simulink library "vhit_control_library"  (R2023a)
settings: Solver=VariableStepAuto  StartTime=0.0  StopTime=10.0  RelTol=1e-3
undefined symbols (not defined in the file): bit, cstElctSpdMaxVal, cstSlowTaskSampTime, parDirCurrMaxVal, parElctSpdMaxVal, parFluxObsFiltCoef, parQdrtCurrMaxVal, parRefSpdFallSlewRate, parRefSpdRisSlewRate, PolePairNum
libraries: lib_conversion x90, lib_square_root x11, lib_dynamic_saturator x9, lib_resettable_unit_delay x2, lib_fault_definiteness x1, lib_angle_mapper x1, lib_cart_to_polar_coor_transformer x1, lib_clarke_transform x1, lib_configurable_parameter x1, lib_current_control_decoupling x1, lib_derating_reference_speed_limiter x1, lib_discrete_time_integrator x1
(part 1 of 3)
settings Model: Creator=CAV2OFO  LastModifiedBy=xiaoqiang.yuan
settings SolverCC: AlgebraicLoopSolver=TrustRegion
settings OptimizationCC: ReuseModelBlockBuffer=off
settings DebuggingCC: UnconnectedInputMsg=warning  UnconnectedOutputMsg=warning  UnconnectedLineMsg=warning
settings ModelReferenceCC: EnableRefExpFcnMdlSchedulingChecks=on
settings RTWCC: DLArmComputeVersion=19.05

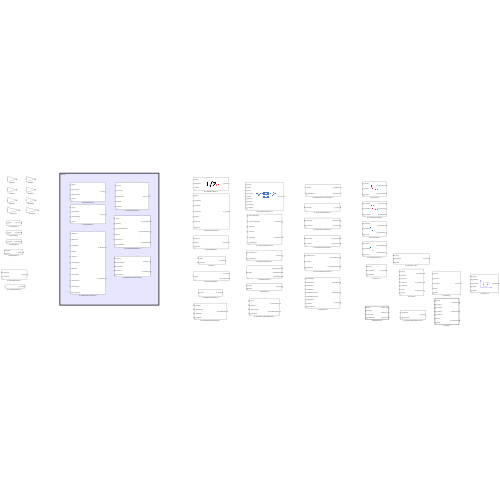
[thumbnail: Simulink's stored preview of the top-level diagram]
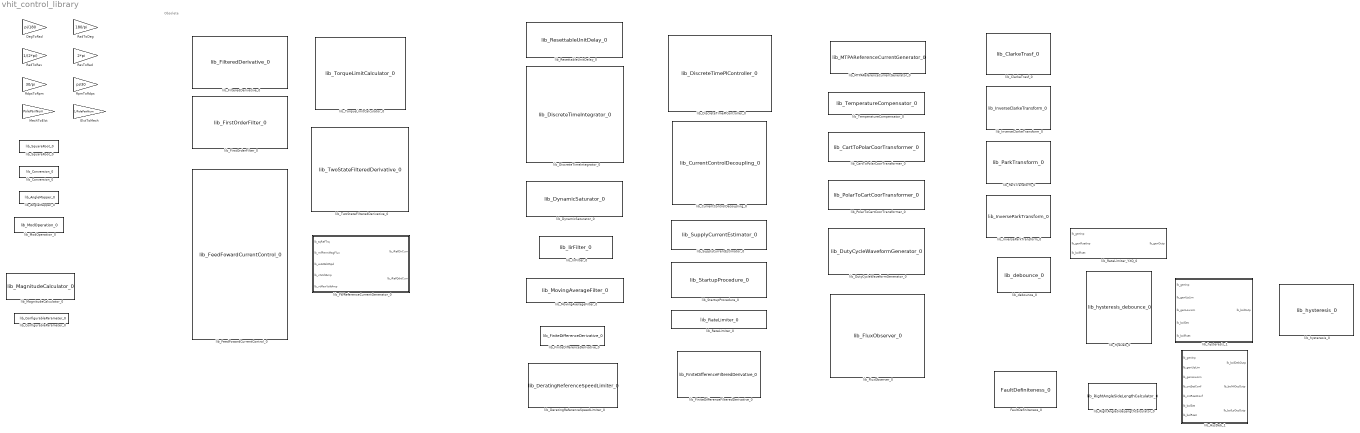
== system vhit_control_library ==
  note: Obsolete
  DegToRad : Gain  Gain=pi/180
  ElctToMech : Gain  Gain=1/PolePairNum
  FaultDefiniteness_0 : lib_fault_definiteness/FaultDefiniteness_0  lb_FaltWaitRecvCnt=0
      link override Constant0: Value=lb_FailWaitRecvCnt
  MechToElct : Gain  Gain=PolePairNum
  RadToDeg : Gain  Gain=180/pi
  RadToRev : Gain  Gain=1/(2*pi)
  RdpsToRpm : Gain  Gain=30/pi
  RevToRad : Gain  Gain=2*pi
  RpmToRdps : Gain  Gain=pi/30
  lib_AngleMapper_0 : lib_angle_mapper/lib_AngleMapper_0  lb_parSlctMappMode=[0,4pi] to [0,2pi]  lb_parOutpDataType=Inherit: Inherit via back propagation
  lib_CartToPolarCoorTransformer_0 : lib_cart_to_polar_coor_transformer/lib_CartToPolarCoorTransformer_0  lb_parAsinLktSize=4095  lb_parAmpLktSize=512  lb_parOutpAmpDataType=fixdt(0,16,2^-10,0)
  lib_ClarkeTrasf_0 : lib_clarke_transform/lib_ClarkeTrasf_0  VariantControl=ClarkTransf_MIL_flo  lb_parAccmDataType=fixdt(1,16,2^-6,0)  lb_parUnBalcSys=off
  lib_ConfigurableParameter_0 : lib_configurable_parameter/lib_ConfigurableParameter_0  lb_parCnfgPar=1  lb_parDataType=Inherit: Inherit from 'Constant value'  lb_parUpLim=2  lb_parLowLim=0
  lib_Conversion_0 : lib_conversion/lib_Conversion_0  lb_parDataType=Inherit: Inherit via back propagation  lb_parOutpMaxVal=[]  lb_parOutpMinVal=[]  lb_parSatFlag=off
  lib_CurrentControlDecoupling_0 : lib_current_control_decoupling/lib_CurrentControlDecoupling_0  lb_parDirIndc=0  lb_parQdrtIndc=0  lb_parMaxPhsIndc=0.001  lb_parMaxElctSpd=4096  lb_parMaxPhsCurr=100  lb_parMaxPermMagFlux=0.01  lb_parMaxCtrlPhsVolt=40  lb_parOutpPekPhy=64  lb_parOutpDataType=fixdt(1,16,2^0,0)
  lib_DeratingReferenceSpeedLimiter_0 : lib_derating_reference_speed_limiter/lib_DeratingReferenceSpeedLimiter_0  lb_parSampTime=parSlowTaskSampTime_u16d6b0  lb_parMaxSampTime=0.01  lb_parMaxIntgGain=parRefSpdLimIntgGainMaxVal  lb_parMaxCurrMarg=100  lb_parMinCurrMarg=-1  lb_parMaxElctRefSpd=2600  lb_parIntgScopMode=Integral control  lb_parSatFlag=on  lb_parAccmDataTypeMode=16-bit  lb_parDtiAccmDataTypeMode=Same of output  lb_parRefSpdDataType=fixdt(1,16,2^-3,0)
  lib_DiscreteTimeIntegrator_0 : lib_discrete_time_integrator/lib_DiscreteTimeIntegrator_0  lb_parMaxInpVal=1  lb_parMinInpVal=-1  lb_parMaxSampTime=0.01  lb_parMaxIntgGain=0  lb_parAccmDataTypeMode=Same of output  lb_parOutpDataType=fixdt(1,16,2^-3,0)  lb_parIntgScopMode=Generic signal  lb_parSatFlag=off
  lib_DiscreteTimePIController_0 : lib_discrete_time_PI_controller/lib_DiscreteTimePIController_0  lb_parSampTime=0.01  lb_parMaxSampTime=1  lb_parMaxPropGain=1  lb_parMaxIntgGain=1  lb_parRefInpMaxVal=4096  lb_parRefInpMinVal=-4096  lb_parMaxErrVal=4096*2  lb_parMinErrVal=-4096*2  lb_parMaxOutpVal=20  lb_parMinOutpVal=-20  lb_parAccmDataTypeMode=32-bit  lb_parOutpDataType=fixdt(1,16,2^-14,0)  lb_parSatMode=anti-windup with back-calculation
  lib_DutyCycleWaveformGenerator_0 : lib_duty_cycle_waveform_generator/lib_DutyCycleWaveformGenerator_0  lb_parLktSize=1024  lb_parOmodFact=1  lb_parPWMMode=Sinusoidal plus third harmonics modulation
  lib_DynamicSaturator_0 : lib_dynamic_saturator/lib_DynamicSaturator_0
  lib_FWReferenceCurrentGenerator_0 : Subsystem  mask{lb_parPolePairNum=5, lb_parPermMagFlux=2e-3, lb_parMagTempCoef=-1e-3, lb_parDirIndc=1e-5, lb_parQdrtIndc=1e-5, lb_parMaxPhsCurr=50, lb_parRatSplyVolt=12, lb_parRsrvVolt=0, lb_parDmgzFact=1, lb_parPWMMode=Sinusoidal, lb_parFWEnbl=off, lb_parMaxOperTrq=1, lb_parMinOperTrq=-1, lb_parTrqSampNum=60, lb_parMaxOperTemp=140, lb_parMinOperTemp=-20, lb_parTempSampNum=20, lb_parElctSpdSampNum=40, lb_parOutpDataType=Inherit: Inherit via back propagation}
      mask prompts: lb_parPolePairNum "Pole pairs number [-]:"; lb_parPermMagFlux "Permanent magnet flux at 20[oC]:"; lb_parMagTempCoef "Magnet temperature coefficient [1/K]:"; lb_parDirIndc "Direct inductance [H]:"; lb_parQdrtIndc "Quadrature inductance [H]:"; lb_parMaxPhsCurr "Maximum phase current [A]:"; lb_parRatSplyVolt "Rated supply voltage [V]:"; lb_parRsrvVolt "Reserve voltage [V]:"; lb_parDmgzFact "Demagnetization factor [-]:"; lb_parPWMMode "Pulse width modulation method:"; lb_parFWEnbl "Field weakening strategy"; lb_parMaxOperTrq "Maximum operating torque [Nm]:"; lb_parMinOperTrq "Minimum operating torque [Nm]:"; lb_parTrqSampNum "Torque samplings number:"; lb_parMaxOperTemp "Maximum operating temperature [oC]:"; lb_parMinOperTemp "Minimum operating temperature [oC]:"; lb_parTempSampNum "Temperature samplings number:"; lb_parElctSpdSampNum "Electric angular speed samplings number:"; lb_parOutpDataType "Output data type:"
      mask init:
      | if lb_parFWEnbl
      |     set_param([gcb,'/vss_ActiveReferenceCurrentStrategy'],'LabelModeActiveChoice','lb_parFWStrgLbl');
      | else
      |     set_param([gcb,'/vss_ActiveReferenceCurrentStrategy'],'LabelModeActiveChoice','lb_parMTPAStrgLbl');
      | end
      | 
      | temp.PermMagFlux_scl = double(lb_parPermMagFlux);  % [Vs] Permanent magnet flux at 20°C
      | temp.Ld_scl = double(lb_parDirIndc);  % [H] Direct inductance
      | temp.Lq_scl = double(lb_parQdrtIndc);  % [H] Quadrature inductance
      | temp.Npp_scl = double(lb_parPolePairNum);  % Number of pole pairs
      | temp.TmpCoeff_scl = double(lb_parMagTempCoef);  % [1/K] Temperature coefficient of permanent magnet
      | temp.DCVolt_scl = double(lb_parRatSplyVolt);  % [V] Rated supply voltage
      | temp.ResVolt_scl = double(lb_parRsrvVolt);  % [V] Reserve voltage from limit condition
      | temp.IPhaseMax_scl = double(lb_parMaxPhsCurr);  % [A] Max phase current
      | 
      | % Limit voltage depending on PWM strategy
      | temp.MaxVolt_scl = temp.DCVolt_scl/2;
      | switch lb_parPWMMode
      |     case 'Sinusoidal'
      |         temp.MaxVolt_scl = temp.DCVolt_scl/2;
      |     case 'Sinusoidal plus third harmonics'
      |         temp.MaxVolt_scl = temp.DCVolt_scl/sqrt(3);
      |     case 'Space vector modulation'
      |         temp.MaxVolt_scl = temp.DCVolt_scl/sqrt(3);
      |     case 'Discontinuous minimum PWM'
      |         temp.MaxVolt_scl = temp.DCVolt_scl/sqrt(3);
      | end
      | lb_parMaxVolt = temp.MaxVolt_scl;
      | 
      | lb_parRatSplyVoltLimCoef = 0.2;  % Max under/over supply voltage w.r.t. rated supply voltage
      | 
      | % Define torque data
      | temp.Trq_arr = linspace(lb_parMinOperTrq,lb_parMaxOperTrq,lb_parTrqSampNum);  % [Nm] Reference values of electric torque
      | temp.NewTrqStep_scl = 2^(ceil(log2((lb_parMaxOperTrq-lb_parMinOperTrq)/(lb_parTrqSampNum-1))));
      | temp.NewMaxTrq_scl = lb_parMinOperTrq + temp.NewTrqStep_scl*(lb_parTrqSampNum-1);
      | temp.Trq_arr = (lb_parMinOperTrq:temp.NewTrqStep_scl:temp.NewMaxTrq_scl);
      | 
      | % Define temperature/permanent magnet flux data
      | temp.MaxPermMagFlux_scl = temp.PermMagFlux_scl*(1+temp.TmpCoeff_scl*(lb_parMinOperTemp-20));
      | temp.MinPermMagFlux_scl = temp.PermMagFlux_scl*(1+temp.TmpCoeff_scl*(lb_parMaxOperTemp-20));
      | temp.PermMagFlux_arr = linspace(temp.MinPermMagFlux_scl,temp.MaxPermMagFlux_scl,lb_parTempSampNum);
      | temp.NewPermMagFluxStep_scl = 2^(ceil(log2((temp.MaxPermMagFlux_scl-temp.MinPermMagFlux_scl)/(lb_parTempSampNum-1))));
      | temp.NewMaxPermMagFlux_scl = temp.MinPermMagFlux_scl + temp.NewPermMagFluxStep_scl*(lb_parTempSampNum-1);
      | temp.PermMagFlux_arr = linspace(temp.MinPermMagFlux_scl,temp.NewMaxPermMagFlux_scl,lb_parTempSampNum);
      | 
      | temp.IdMTPA_mat = zeros(lb_parTrqSampNum,lb_parTempSampNum);  % [A] Initialization of MTPA LUT
      | 
      | if lb_parFWEnbl
      |     
      |     % Base speed
      |     temp.IdLim_arr = temp.PermMagFlux_arr/4/(temp.Lq_scl-temp.Ld_scl) + ...
      |         - sqrt((temp.PermMagFlux_arr/4/(temp.Lq_scl-temp.Ld_scl)).^2 + temp.IPhaseMax_scl^2/2);
      |     temp.IqLim_arr = sqrt(temp.IPhaseMax_scl^2 - temp.IdLim_arr.^2);
      |     temp.BaseSpd_arr = (temp.MaxVolt_scl-temp.ResVolt_scl)./sqrt((temp.Ld_scl*temp.IdLim_arr+temp.PermMagFlux_arr).^2 + ...
      |         (temp.Lq_scl*temp.IqLim_arr).^2);
      |     
      |     % Define electric angular speed data for field weakening control strategy
      |     temp.MinElctSpd_scl = min(temp.BaseSpd_arr)*0.7;  % [rad/s] Minimum electric speed
      |     temp.MaxElctSpd_scl = min(temp.BaseSpd_arr)+1000;  % [rad/s] Maximum electric speed
      |     temp.ElctSpd_arr = linspace(temp.MinElctSpd_scl,temp.MaxElctSpd_scl,lb_parElctSpdSampNum);  % [rad/s] Reference values of electric speed
      |     temp.IdFW_mat = zeros(lb_parTrqSampNum,lb_parTempSampNum,lb_parElctSpdSampNum); % [A] Initialization of FW LUT
      | 
      |     for ii = 1:lb_parTrqSampNum
      |         
      |         for jj = 1:lb_parTempSampNum
      |             
      |             % The following quartic equation represents the Maximum Torque Per Ampere
      |             % control strategy. The solution returns the direct current adsdsadsdds
      |             % corresponding to a given electric torque.
      |             
      |             temp.idMTPA_fun = @(id) 1e10*(9*temp.Npp_scl^2*(temp.Lq_scl-temp.Ld_scl)^3*id.^4 + ...
      |                 - 27*temp.Npp_scl^2*temp.PermMagFlux_arr(jj)*(temp.Lq_scl-temp.Ld_scl)^2*id.^3 + ...
      |                 27*temp.Npp_scl^2*temp.PermMagFlux_arr(jj)^2*(temp.Lq_scl-temp.Ld_scl)*id.^2 + ...
      |                 - 9*temp.Npp_scl^2*temp.PermMagFlux_arr(jj)^3*id + ...
      |                 - 4*(temp.Lq_scl-temp.Ld_scl)*temp.Trq_arr(ii)^2);
      |             
      |             if jj == 1 || jj == 2
      |                 temp.IdMTPA_mat(ii,jj) = real(fzero(temp.idMTPA_fun,-1e-1));
      |             else
      |                 temp.IdMTPA_mat(ii,jj) = fzero(temp.idMTPA_fun,temp.IdMTPA_mat(ii,jj-1));
      |             end
      |             
      |             for kk = 1:lb_parElctSpdSampNum
      |                 
      |                 % The following quartic equation represents the Field Weakening
      |                 % control strategy. The solution returns the direct current
      |                 % corresponding to a given electric torque.
      |                 %                 + temp.PermMagFlux_arr(jj)^2*(temp.Ld_scl^2-4*(temp.Lq_scl-temp.Ld_scl)*temp.Ld_scl + ...
      |                 
      |                 temp.idFW_fun = @(id) 1e12*((temp.Lq_scl-temp.Ld_scl)^2*temp.Ld_scl^2*id.^4 + ...
      |                     + 2*temp.PermMagFlux_arr(jj)*(temp.Lq_scl-temp.Ld_scl)*temp.Ld_scl*(temp.Lq_scl-temp.Ld_scl-temp.Ld_scl)*id.^3 + ...
      |                     + (temp.PermMagFlux_arr(jj)^2*(temp.Ld_scl^2-4*(temp.Lq_scl-temp.Ld_scl)*temp.Ld_scl) + ...
      |                     + (temp.Lq_scl-temp.Ld_scl)^2*(temp.PermMagFlux_arr(jj)^2-(temp.MaxVolt_scl-temp.ResVolt_scl)^2/temp.ElctSpd_arr(kk)^2))*id.^2 + ...
      |                     + 2*temp.PermMagFlux_arr(jj)*(temp.PermMagFlux_arr(jj)^2*(temp.Ld_scl-(temp.Lq_scl-temp.Ld_scl))+...
      |                     + (temp.Lq_scl-temp.Ld_scl)*(temp.MaxVolt_scl-temp.ResVolt_scl)^2/temp.ElctSpd_arr(kk)^2)*id + ...
      |                     + temp.PermMagFlux_arr(jj)^2*(temp.PermMagFlux_arr(jj)^2-(temp.MaxVolt_scl-temp.ResVolt_scl)^2/temp.ElctSpd_arr(kk)^2) + ...
      |                     + 4/9*temp.Lq_scl^2/temp.Npp_scl^2*temp.Trq_arr(ii)^2);
      |                 
      |                 if kk == 1 || kk == 2
      |                     temp.IdFW_mat(ii,jj,kk) = real(fzero(temp.idFW_fun,-1e-1));
      |                 else
      |                     temp.IdFW_mat(ii,jj,kk) = fzero(temp.idFW_fun,temp.IdFW_mat(ii,jj,kk-1));
      |                 end
      |                 
      |             end
      |         end
      |     end
      |     
      |     lb_parMTPATrqData = temp.Trq_arr;
      |     lb_parMTPAPermMagFluxData = temp.PermMagFlux_arr;
      |     lb_parMTPA2DLktMtrx = temp.IdMTPA_mat;
      |     lb_parFWTrqData = temp.Trq_arr;
      |     lb_parFWPermMagFluxData = temp.PermMagFlux_arr;
      |     lb_parFWElctSpdData = temp.ElctSpd_arr;
      |     lb_parFW3DLktMtrx = temp.IdFW_mat;
      |     
      | else
      |     
      |     for ii = 1:lb_parTrqSampNum
      |         
      |         for jj = 1:lb_parTempSampNum
      |             
      |             % The following quartic equation represents the Maximum Torque Per Ampere
      |             % control strategy. The solution returns the direct current adsdsadsdds
      |             % corresponding to a given electric torque.
      |             
      |             temp.idMTPA_fun = @(id) 1e10*(9*temp.Npp_scl^2*(temp.Lq_scl-temp.Ld_scl)^3*id.^4 + ...
      |                 - 27*temp.Npp_scl^2*temp.PermMagFlux_arr(jj)*(temp.Lq_scl-temp.Ld_scl)^2*id.^3 + ...
      |                 27*temp.Npp_scl^2*temp.PermMagFlux_arr(jj)^2*(temp.Lq_scl-temp.Ld_scl)*id.^2 + ...
      |                 - 9*temp.Npp_scl^2*temp.PermMagFlux_arr(jj)^3*id + ...
      |                 - 4*(temp.Lq_scl-temp.Ld_scl)*temp.Trq_arr(ii)^2);
      |             
      |             if jj == 1 || jj == 2
      |                 temp.IdMTPA_mat(ii,jj) = real(fzero(temp.idMTPA_fun,-1e-1));
      |             else
      |                 temp.IdMTPA_mat(ii,jj) = fzero(temp.idMTPA_fun,temp.IdMTPA_mat(ii,jj-1));
      |             end
      |             
      |         end
      |     end
      |     
      |     lb_parMTPATrqDataFrstVal = temp.Trq_arr(1);
      |     lb_parMTPATrqDataStepVal = temp.NewTrqStep_scl;
      |     lb_parMTPAPermMagFluxDataFrstVal = temp.PermMagFlux_arr(1);
      |     lb_parMTPAPermMagFluxDataStepVal = temp.NewPermMagFluxStep_scl;
      |     lb_parMTPA2DLktMtrx = temp.IdMTPA_mat;
      |     
      | end
      | 
      | clear temp
      settings: LibrarySourceBlock=lib_reference_current_generator/lib_ReferenceCurrentGenerator_0
      mask TypeOptions lb_parPWMMode: Sinusoidal | Sinusoidal plus third harmonics | Space vector modulation | Discontinuous minimum PWM
      mask DialogControl DescGroupVar Prompt: VHIT control library
      mask DialogControl DescTextVar Prompt: Reference current generator
      mask DialogControl Container4 Prompt: Lookup table parameters
      mask DialogControl Container3 Prompt: Data type
  lib_FeedFowardCurrentControl_0 : lib_feed_foward_current_control/lib_FeedFowardCurrentControl_0  lb_parDirCurrMaxVal=parDirCurrMaxVal  lb_parDirCurrMinVal=-parDirCurrMaxVal  lb_parQdrtCurrMaxVal=parQdrtCurrMaxVal  lb_parQdrtCurrMinVal=-parQdrtCurrMaxVal  lb_parElctSpdMaxVal=parElctSpdMaxVal  lb_parElctSpdMinVal=-parElctSpdMaxVal  lb_parDirIndcMaxVal=parDirIndcMaxVal  lb_parQdrtIndcMaxVal=parQdrtIndcMaxVal  lb_parPhsRsntMaxVal=parPhsRstnMaxVal  lb_parPermMagFluxMaxVal=parPermMagFluxMaxVal  lb_parOutpDataType=fixdt(1,16,2^-9,0)
  lib_FilteredDerivative_0 : lib_filtered_derivative/lib_FilteredDerivative_0  lb_parSampTime=5e-4  lb_parTimeCnst=1e-3  lb_parMaxTimeCnst=1e-1  lb_parMinTimeCnst=1e-4  lb_parMaxOutpVal=1  lb_parAngInpMode=on  lb_parIIntrDataTypeMode=Same of output  lb_parOutpDataType=fixdt(1,16,2^-3,0)
      link override lib_TimeCnst_1: SourceBlock=vhit_control_library/lib_ConfigurableParameter_0
      link override lib_TimeCnst_2: SourceBlock=vhit_control_library/lib_ConfigurableParameter_0
  lib_FiniteDifferenceDerivative_0 : lib_finite_difference_derivative/lib_FiniteDifferenceDerivative_0  lb_parSampTime=0.01  lb_parMaxInpVar=0.1  lb_parOutpPhyPek=4096  lb_parAngInpMode=on  lb_parOutpDataType=fixdt(1,16,2^0,0)
  lib_FiniteDifferenceFilteredDerivative_0 : lib_finite_difference_filtered_derivative/lib_FiniteDifferenceFilteredDerivative_0  lb_parSampTime=0  lb_parInpMaxVal=100  lb_parInpEstErrMaxVal=0.1  lb_parInpDiffMaxVal=0.5  lb_parMaxEstErrCompFreq=4000  lb_parFltrCoefMaxVal=0.3  lb_genOutpUpLim=0  lb_genOutpLowLim=0  lb_parOutpPekPhy=4096  lb_parAngInpMode=on  lb_parOutpDataType=fixdt(1,16,0)
  lib_FirstOrderFilter_0 : lib_first_order_filter/lib_FirstOrderFilter_0  lb_parSampTime=0.01  lb_parTimeCnst=0.001  lb_parMaxTimeCnst=0  lb_parMinTimeCnst=0  lb_parMaxInpVal=1  lb_parInpVrntMaxVal=0  lb_parAccmDataType=fixdt(1,32,2^-25,0)  lb_parIIntrDataTypeMode=Same of output  lb_parOutpDataType=fixdt(1,16,2^-3,0)
  lib_FluxObserver_0 : lib_flux_observer/lib_FluxObserver_0  lb_parPhsIndc=parDirIndc_u16p29b0  lb_parPhsRstnMaxVal=parPhsRstnMaxVal  lb_parPhsIndcMaxVal=parPhsRstnMaxVal  lb_parPhsCurrMaxVal=parPhsCurrMaxVal  lb_parPhsVoltMaxVal=parPhsVoltMaxVal  lb_parEstMagFluxMaxVal=0.01  lb_parPolePairNum=parPolePairNum_u8n0b0  lb_parSampTime=parFastTaskSampTime_u16d6b0  lb_parFltrCoefMaxVal=double(parFluxObsFiltCoef)  lb_parFiltCoef=parFluxObsFiltCoef  lb_parFluxDataType=fixdt(0,16,2^-22,0)  lb_parMotTrqDataType=fixdt(1,16,2^-14,0)  lb_parBitNumMode=32-bit
  lib_HysDeb_0 : lib_hysteresis_debounce/lib_hysteresis_debounce_0  lb_parInitOutp=0
  lib_HysDeb_1 : Subsystem  TreatAsAtomicUnit=on  RTWFcnName=HysteresisDebounce  RTWFileName=VHIT_control_library  mask{lb_parInitOutp=0}
      mask prompts: lb_parInitOutp "Initialization value"
      settings: RTWFcnNameOpts=User specified
      mask DialogControl DescGroupVar Prompt: WEIFU Motor Control Library
      mask DialogControl DescTextVar Prompt: Hysteresis and Debounce
      mask DialogControl ParameterGroupVar Prompt: 参数
  lib_IirFilter_0 : lib_iir_filter/lib_IirFilter_0  lb_parMaxInpVal=2000  lb_parFltrCoefMaxVal=0.02  lb_parBitNumMode=16-bit  lb_parOutpDataType=fixdt(1,16,2^0,0)  lb_parFiltTypeMode=Low-pass
  lib_InverseClarkeTransform_0 : lib_inverse_clarke_transform/lib_InverseClarkeTransform_0  VariantControl=ClarkTransf_MIL_flo  lb_parSymMot=off
  lib_InverseParkTransform_0 : lib_inverse_park_transform/lib_InverseParkTransform_0  VariantControl=ClarkTransf_MIL_flo  lb_parSelRotFrmeAxis=d-axis
  lib_MTPAReferenceCurrentGenerator_0 : lib_mtpa_reference_current_generator/lib_MTPAReferenceCurrentGenerator_0  lb_parPolePairNum=5  lb_parPermMagFlux=2e-3  lb_parMagTempCoef=-1e-3  lb_parDirIndc=1e-5  lb_parQdrtIndc=1e-5  lb_parMaxPhsCurr=50  lb_parDmgzFact=1  lb_parMaxOperTrq=1  lb_parMinOperTrq=-1  lb_parTrqSampNum=60  lb_parMaxOperTemp=140  lb_parMinOperTemp=-20  lb_parTempSampNum=20  lb_parOutpDataType=Inherit: Inherit via back propagation
      settings: LibrarySourceBlock=lib_reference_current_generator/lib_ReferenceCurrentGenerator_0
  lib_MagnitudeCalculator_0 : lib_magnitude_calculator/lib_MagnitudeCalculator_0  lb_parLktSize=512  lb_parOutpDataType=Inherit: Inherit via back propagation
  lib_ModOperation_0 : lib_mod_operation/lib_ModOperation_0  lb_parOutpDataType=Inherit: Inherit via back propagation
  lib_MovingAverageFilter_0 : lib_moving_average_filter/lib_MovingAverageFilter_0  lb_parSampNum=10  lb_parInpSmtnDataType=fixdt(1,32,2^-19,0)
  lib_ParkTransform_0 : lib_park_transform/lib_ParkTransform_0  VariantControl=ClarkTransf_MIL_flo  lb_parSelRotFrmeAxis=d-axis
  lib_PolarToCartCoorTransformer_0 : lib_polar_to_cart_coor_transformer/lib_PolarToCartCoorTransformer_0  lb_parLktSize=1024  lb_parOutpDataType=Inherit: Inherit via back propagation
  lib_RateLimiter_0 : lib_rate_limiter/lib_RateLimiter_0  lb_parSampTime=parSlowTaskSampTime_u16d6b0  lb_parRiseSlewRate=parRefSpdRisSlewRate_s16d0b0  lb_parFallSlewRate=parRefSpdFallSlewRate_s16d0b0  lb_parMaxInpVal=parElctSpdMaxVal  lb_parMinInpVal=-parElctSpdMaxVal
  lib_RateLimiter_YXQ_0 : Subsystem  mask{lb_parSampTime=cstSlowTaskSampTime, lb_parRiseSlewRate=parRefSpdRisSlewRate, lb_parFallSlewRate=parRefSpdFallSlewRate, lb_parMaxInpVal=cstElctSpdMaxVal, lb_parMinInpVal=-cstElctSpdMaxVal}
      mask prompts: lb_parSampTime "Sampling time [s]:"; lb_parRiseSlewRate "Rising slew rate:"; lb_parFallSlewRate "Falling slew rate:"; lb_parMaxInpVal "Input signal max value"; lb_parMinInpVal "Input signal min value"
      mask init:
      | %Re-initialize parameters in Double
      | lb_parMaxInpVal = double(lb_parMaxInpVal);
      | lb_parMinInpVal = double(lb_parMinInpVal);
      | lb_parSampTime_temp = double(lb_parSampTime);
      | 
      | % Data type for input variation
      | lb_parInpVrntMaxVal = abs(lb_parMaxInpVal-lb_parMinInpVal);
      | 
      | % Data type for the derivative of the input signal
      | lb_parInpDrvtMaxVal = abs(lb_parMaxInpVal-lb_parMinInpVal)/lb_parSampTime_temp;
      | lb_parInpDrvtDataType = Simulink.NumericType;
      | lb_parInpDrvtDataType.DataTypeMode= 'Fixed-point: unspecified scaling';
      | if lb_parInpDrvtMaxVal <= (2^15)-1
      |     lb_parInpDrvtDataType.WordLength = 16;
      | else
      |     lb_parInpDrvtDataType.WordLength = 32;
      | end
      | 
      | %Min-Max limit for Sampling Time * Rise/Fall Slew rate 
      | lb_parAccmDataTypeMax = double(lb_parSampTime_temp*lb_parRiseSlewRate);
      | lb_parAccmDataTypeMin = double(lb_parSampTime_temp*lb_parFallSlewRate);
      | lb_parAccmDataType_temp = fi([lb_parAccmDataTypeMin lb_parAccmDataTypeMax]);
      | lb_parAccmDataType = Simulink.NumericType;
      | lb_parAccmDataType.DataTypeMode= 'Fixed-point: slope and bias scaling';
      | lb_parAccmDataType.Signedness = lb_parAccmDataType_temp.Signedness;
      | lb_parAccmDataType.WordLength = lb_parAccmDataType_temp.WordLength;
      | lb_parAccmDataType.Slope = 2^(-lb_parAccmDataType_temp.FractionLength);
      | 
      | % lb_parAccmDataType = Simulink.NumericType;
      | % lb_parAccmDataType.DataTypeMode= 'Fixed-point: unspecified scaling';
      | % if lb_parAccmDataTypeMax <= (2^15)-1
      | %     lb_parAccmDataType.WordLength = 16;
      | % else
      | %     lb_parAccmDataType.WordLength = 32;
      | % end
      | 
      | %% Convert to double parameters needed to compute data types
      | 
      | % lb_parRiseSlewRate = double(lb_parRiseSlewRate);
      | % 
      | % %% Define of data type for product u*Ts
      | % % lb_parIntgStepDataTypeMaxVal = lb_parMaxInpVal*lb_parSampTime*lb_parRiseSlewRate;
      | % lb_parOutpDataType = Simulink.NumericType;
      | % lb_parOutpDataType.DataTypeMode= 'Fixed-point: unspecified scaling';
      | % if lb_parMinInpVal < 0
      | %     lb_parOutpDataType.Signedness = 'Signed';
      | %     if lb_parMaxInpVal <= (2^16)/2-1
      | %         lb_parOutpDataType.WordLength = 16;
      | %     else
      | %         lb_parOutpDataType.WordLength = 32;
      | %     end
      | % else
      | %     lb_parOutpDataType.Signedness = 'Unsigned';
      | %         if lb_parMaxInpVal <= (2^16)-1
      | %         lb_parOutpDataType.WordLength = 16;
      | %     else
      | %         lb_parOutpDataType.WordLength = 32;
      | %     end
      | % end
      settings: LibrarySourceBlock=lib_rate_limiter/lib_RateLimiter_0
      mask DialogControl DescGroupVar Prompt: WEIFU Motor Control Libray
      mask DialogControl DescTextVar Prompt: Rate Limiter Block
  lib_ResettableUnitDelay_0 : lib_resettable_unit_delay/lib_ResettableUnitDelay_0
  lib_RightAngleSideLengthCalculator_0 : lib_right_angle_side_length_calculator/lib_RightAngleSideLengthCalculator_0  lb_parLktSize=512  lb_parOutpDataType=Inherit: Inherit via back propagation
  lib_SquareRoot_0 : lib_square_root/lib_SquareRoot_0  lb_parLktSize=128  lb_parInpDataType=uint16  lb_parOutpDataType=Inherit: Inherit via back propagation
  lib_StartupProcedure_0 : lib_startup_procedure/lib_StartupProcedure_0  lb_parSampTime=2e-3  lb_parStrtUpSpdRampCoef=2000  lb_parStrtUpTrqRampCoef=30  lb_parStrtUpSpd=200  lb_parStrtUpTrq=0.6  lb_parSpdRampCoefMaxVal=10000*5*pi/30  lb_parSpdRampCoefMinVal=-10000*5*pi/30  lb_parTrqRampCoefMaxVal=30  lb_parTrqRampCoefMinVal=-30  lb_parMaxSampTime=lb_parSampTime  lb_parMaxIntgGain=0  lb_parIntgScopMode=Generic signal  lb_parSatFlag=on  lb_parSpdAccmDataTypeMode=32-bit  lb_parTrqAccmDataTypeMode=32-bit  lb_parElctSpdDataType=fixdt(1,16,2^0,0)  lb_parTrqDataType=fixdt(1,16,2^0,0)
  lib_SupplyCurrentEstimator_0 : lib_supply_current_estimator/lib_SupplyCurrentEstimator_0  lb_parOutpDataType=Inherit: Inherit via back propagation
  lib_TemperatureCompensator_0 : lib_temperature_compensator/lib_TemperatureCompensator_0  lb_parTempCoef=-1e-3  lb_parRefTemp=20  lb_parRefTempOutpVal=0
  lib_TorqueLimitCalculator_0 : lib_torque_limit_calculator/lib_TorqueLimitCalculator_0  lb_parSampTime=0.01  lb_parMaxSampTime=0.01  lb_parIntgGain=0  lb_parMaxIntgGain=1  lb_parMaxInpVal=50  lb_parMinInpVal=-1  lb_parIntgScopMode=Integral control  lb_parSatFlag=on  lb_parAccmDataTypeMode=32-bit  lb_parOutpDataType=fixdt(1,16,2^-14,0)
  lib_TwoStateFilteredDerivative_0 : lib_two_state_filtered_derivative/lib_TwoStateFilteredDerivative_0  lb_parSampTime=parMedTaskSampTime_u16d6b0  lb_parMaxSampTime=lb_parMaxSampTime  lb_parMaxCharFreq=parSpdDrvtCharFreqMaxVal  lb_parMaxDampCoef=parSpdDrvtDampCoefMaxVal  lb_parIntgMaxInpVal=lb_parMaxSampTime  lb_parIntgMinInpVal=lb_parMaxSampTime  lb_genFstStatOutpUpLim=parElctSpdMaxVal  lb_genFstStatOutpLowLim=-parElctSpdMaxVal  lb_genInpEstErrMaxVal=parElctAngEstMaxVal  lb_parAngInpMode=on  lb_parAccmDataTypeMode=32-bit  lb_parFstStatOutpDataType=fixdt(1,16,2^-3,0)  lb_parSndStatOutpDataType=fixdt(1,16,2^0,0)  lb_parIntgScopMode=Integral control  lb_parSatFlag=on
  lib_debounce_0 : lib_debounce/lib_debounce_0
  lib_hysteresis_0 : lib_hysteresis/lib_hysteresis_0
  lib_hysteresis_1 : Subsystem  RTWFcnName=Hysteresis  RTWFileName=VHIT_control_library  mask{lb_parInitOutp=0}
      mask prompts: lb_parInitOutp "Initial Parameter"
      settings: RTWFcnNameOpts=User specified
      mask DialogControl DescGroupVar Prompt: WF Motor Control Library
      mask DialogControl DescTextVar Prompt: Hysteresis
      mask DialogControl ParameterGroupVar Prompt: 参数

== system vhit_control_library/lib_FWReferenceCurrentGenerator_0 ==
  lb_tqRefTrq : Inport
  lb_mfPermMagFlux : Inport  Port=2
  lb_wActElctSpd : Inport  Port=3
  lb_vtVoltAmp : Inport  Port=4
  lb_vtMaxVoltAmp : Inport  Port=5
  vss_ActiveReferenceCurrentStrategy : Subsystem  Variant=on  VariantControlMode=label  VariantControl=Variant2  LabelModeActiveChoice=lb_parMTPAStrgLbl
  lb_iRefDirCurr : Outport
  lb_iRefQdrtCurr : Outport  Port=2
  wires:
  lb_vtVoltAmp/1 -> vss_ActiveReferenceCurrentStrategy/4(lb_vtVoltAmp)
  vss_ActiveReferenceCurrentStrategy/2(lb_iRefQdrtCurr) -> lb_iRefQdrtCurr/1
  vss_ActiveReferenceCurrentStrategy/1(lb_iRefDirCurr) -> lb_iRefDirCurr/1
  lb_tqRefTrq/1 -> vss_ActiveReferenceCurrentStrategy/1(lb_tqRefTrq)
  lb_wActElctSpd/1 -> vss_ActiveReferenceCurrentStrategy/3(lb_wActElctSpd)
  lb_mfPermMagFlux/1 -> vss_ActiveReferenceCurrentStrategy/2(lb_mfPermMagFlux)
  lb_vtMaxVoltAmp/1 -> vss_ActiveReferenceCurrentStrategy/5(lb_vtMaxVoltAmp)

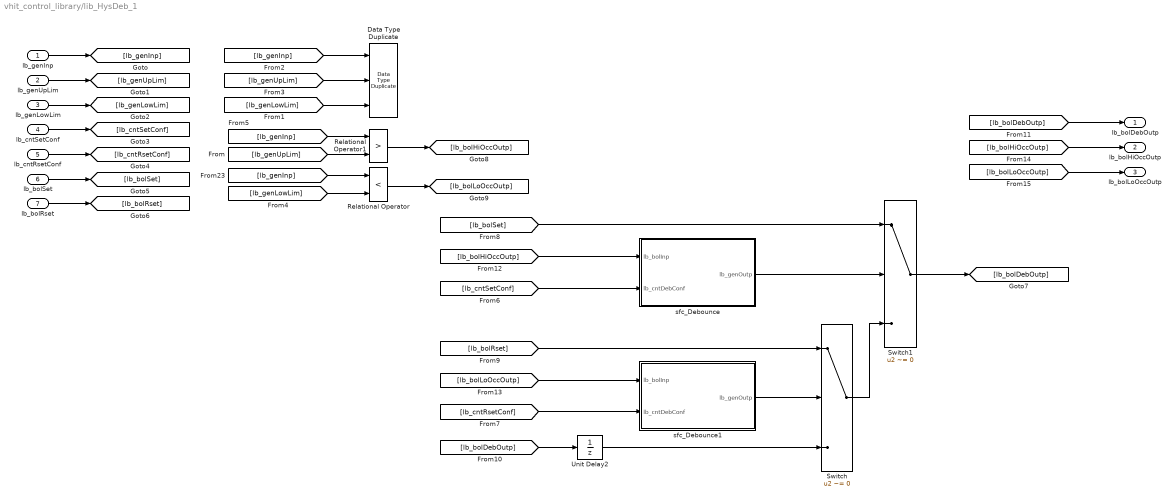
== system vhit_control_library/lib_HysDeb_1 ==
  lb_genInp : Inport
  lb_genUpLim : Inport  Port=2
  lb_genLowLim : Inport  Port=3
  lb_cntSetConf : Inport  Port=4
  lb_cntRsetConf : Inport  Port=5
  lb_bolSet : Inport  Port=6
  lb_bolRset : Inport  Port=7
  Data Type Duplicate : DataTypeDuplicate  NumInputPorts=3
  Relational Operator : RelationalOperator  Operator=<  OutDataTypeStr=boolean  InputSameDT=off
  Relational Operator1 : RelationalOperator  Operator=>  OutDataTypeStr=boolean  InputSameDT=off
  Switch : Switch  Criteria=u2 ~= 0  SaturateOnIntegerOverflow=off  InputSameDT=off  OutDataTypeStr=Inherit: Same as first input
  Switch1 : Switch  Criteria=u2 ~= 0  SaturateOnIntegerOverflow=off  InputSameDT=off  OutDataTypeStr=Inherit: Same as first input
  Unit Delay2 : UnitDelay  InitialCondition=lb_parInitOutp  SampleTime=-1  HasFrameUpgradeWarning=on
  sfc_Debounce : Stateflow chart  TreatAsAtomicUnit=on
  sfc_Debounce1 : Stateflow chart  TreatAsAtomicUnit=on
  lb_bolDebOutp : Outport
  lb_bolHiOccOutp : Outport  Port=2
  lb_bolLoOccOutp : Outport  Port=3
  wires:
  [lb_bolLoOccOutp] -> lb_bolLoOccOutp/1
  [lb_bolHiOccOutp] -> lb_bolHiOccOutp/1
  [lb_bolLoOccOutp] -> sfc_Debounce1/1(lb_bolInp)
  [lb_bolHiOccOutp] -> sfc_Debounce/1(lb_bolInp)
  Relational Operator/1 -> [lb_bolLoOccOutp]
  Relational Operator1/1 -> [lb_bolHiOccOutp]
  [lb_bolDebOutp] -> lb_bolDebOutp/1
  [lb_bolSet] -> Switch1/1
  [lb_bolRset] -> Switch/1
  [lb_cntRsetConf] -> sfc_Debounce1/2(lb_cntDebConf)
  Switch/1 -> Switch1/3
  sfc_Debounce1/1(lb_genOutp) -> Switch/2
  [lb_bolDebOutp] -> Unit Delay2/1
  Unit Delay2/1 -> Switch/3
  lb_bolRset/1 -> [lb_bolRset]
  sfc_Debounce/1(lb_genOutp) -> Switch1/2
  lb_bolSet/1 -> [lb_bolSet]
  lb_cntRsetConf/1 -> [lb_cntRsetConf]
  lb_cntSetConf/1 -> [lb_cntSetConf]
  [lb_genInp] -> Relational Operator1/1
  [lb_genLowLim] -> Data Type Duplicate/3
  [lb_genUpLim] -> Data Type Duplicate/2
  [lb_genInp] -> Data Type Duplicate/1
  lb_genLowLim/1 -> [lb_genLowLim]
  lb_genUpLim/1 -> [lb_genUpLim]
  lb_genInp/1 -> [lb_genInp]
  [lb_cntSetConf] -> sfc_Debounce/2(lb_cntDebConf)
  [lb_genUpLim] -> Relational Operator1/2
  Switch1/1 -> [lb_bolDebOutp]
  [lb_genInp] -> Relational Operator/1
  [lb_genLowLim] -> Relational Operator/2

== system vhit_control_library/lib_RateLimiter_YXQ_0 ==
  lb_genInp : Inport
  lb_genRsetInp : Inport  Port=2
  lb_bolRset : Inport  Port=3
  Chart : Stateflow chart  TreatAsAtomicUnit=on
  Subsystem : Subsystem
  Switch : Switch  Criteria=u2 ~= 0  SaturateOnIntegerOverflow=off  InputSameDT=off
  Terminator : Terminator
  sss_DecrementFlagTrigger : Subsystem
  sss_IncrementFlagTrigger : Subsystem
  lb_genOutp : Outport
  wires:
  Switch/1 -> [lb_genOutp]
  Subsystem/1(lb_genIncrOutp) -> [lb_genIncrOutp]
  [lb_bolRset] -> Subsystem/4(lb_bolRset)
  lb_genRsetInp/1 -> [lb_genRsetInp]
  lb_genInp/1 -> [lb_genInp]
  [lb_genInp] -> sss_IncrementFlagTrigger/1(lb_genInp)
  sss_IncrementFlagTrigger/1(lb_incrRatLimOn) -> [lb_incrRatLimOn]
  sss_DecrementFlagTrigger/1(lb_decrRatLimOn) -> [lb_decrRatLimOn]
  [lb_genDelyOutp] -> sss_DecrementFlagTrigger/2(lb_genDelyOutp)
  [lb_genInp] -> sss_DecrementFlagTrigger/1(lb_genInp)
  [lb_incrRatLimOn] -> Chart/1(lb_incrRatLimOn)
  [lb_decrRatLimOn] -> Chart/2(lb_decrRatLimOn)
  Chart/1(lb_noRatLimReq) -> [lb_noRatLimReq]
  Chart/2(lb_incrRatLimReq) -> [lb_incrRatLimReq]
  Chart/3(lb_decrRatLimReq) -> Terminator/1
  [lb_genRsetInp] -> Subsystem/1(lb_genInp)
  [lb_genOutp] -> lb_genOutp/1
  Subsystem/2(lb_genDelyOutp) -> [lb_genDelyOutp]
  [lb_genDelyOutp] -> sss_IncrementFlagTrigger/2(lb_genDelyOutp)
  [lb_incrRatLimReq] -> Subsystem/3(lb_incrRatLimReq)
  [lb_noRatLimReq] -> Subsystem/2(lb_noRatLimReq)
  [lb_genIncrOutp] -> Switch/3
  [lb_noRatLimReq] -> Switch/2
  [lb_genInp] -> Switch/1
  lb_bolRset/1 -> [lb_bolRset]

== system vhit_control_library/lib_hysteresis_1 ==
  lb_genInp : Inport
  lb_genUpLim : Inport  Port=2
  lb_genLowLim : Inport  Port=3
  lb_bolSet : Inport  Port=4
  lb_bolRset : Inport  Port=5
  Data Type Duplicate : DataTypeDuplicate  NumInputPorts=3
  Relational Operator : RelationalOperator  Operator=<  OutDataTypeStr=boolean  InputSameDT=off
  Relational Operator1 : RelationalOperator  Operator=>  OutDataTypeStr=boolean  InputSameDT=off
  Switch : Switch  Criteria=u2 ~= 0  SaturateOnIntegerOverflow=off  InputSameDT=off  OutDataTypeStr=Inherit: Same as first input
  Switch1 : Switch  Criteria=u2 ~= 0  SaturateOnIntegerOverflow=off  InputSameDT=off  OutDataTypeStr=Inherit: Same as first input
  Unit Delay2 : UnitDelay  InitialCondition=lb_parInitOutp  SampleTime=-1  HasFrameUpgradeWarning=on
  lb_bolOutp : Outport
  wires:
  lb_genUpLim/1 -> Relational Operator1/2, Data Type Duplicate/3
  Switch1/1 -> lb_bolOutp/1, Unit Delay2/1
  Unit Delay2/1 -> Switch/3
  lb_genInp/1 -> Relational Operator/1, Relational Operator1/1, Data Type Duplicate/1
  lb_genLowLim/1 -> Relational Operator/2, Data Type Duplicate/2
  lb_bolSet/1 -> Switch1/1
  lb_bolRset/1 -> Switch/1
  Relational Operator/1 -> Switch/2
  Relational Operator1/1 -> Switch1/2
  Switch/1 -> Switch1/3

== system vhit_control_library/lib_FWReferenceCurrentGenerator_0/vss_ActiveReferenceCurrentStrategy ==
  lb_tqRefTrq : Inport
  lb_mfPermMagFlux : Inport  Port=2
  lb_wActElctSpd : Inport  Port=3
  lb_vtVoltAmp : Inport  Port=4
  lb_vtMaxVoltAmp : Inport  Port=5
  vss_FieldWeakeningStrategy : Subsystem  VariantControl=lb_parFWStrgLbl
  vss_MaximumTorquePerAmpereStrategy : Subsystem  VariantControl=lb_parMTPAStrgLbl
  lb_iRefDirCurr : Outport  VectorParamsAs1DForOutWhenUnconnected=off
  lb_iRefQdrtCurr : Outport  Port=2  VectorParamsAs1DForOutWhenUnconnected=off

== system vhit_control_library/lib_RateLimiter_YXQ_0/Subsystem ==
  lb_genInp : Inport
  lb_noRatLimReq : Inport  Port=2
  lb_incrRatLimReq : Inport  Port=3
  lb_bolRset : Inport  Port=4
  Add1 : Sum  OutDataTypeStr=Inherit: Inherit via back propagation  RndMeth=Simplest
  Constant : Constant  Value=0  OutDataTypeStr=Inherit: Inherit via back propagation  LockScale=on
  Constant1 : Constant  Value=lb_parFallSlewRate
  Constant2 : Constant  Value=lb_parRiseSlewRate
  Constant4 : Constant  Value=lb_parSampTime
  Data Type Duplicate : DataTypeDuplicate
  Data Type Duplicate1 : DataTypeDuplicate  NumInputPorts=3
  Data Type Conversion : DataTypeConversion  OutDataTypeStr=lb_parAccmDataType  RndMeth=Simplest  SaturateOnIntegerOverflow=off
  Data Type Conversion1 : DataTypeConversion  Commented=on  OutMin=lb_parMinInpVal  OutMax=lb_parMaxInpVal  OutDataTypeStr=fixdt(1,32)  SaturateOnIntegerOverflow=off  RndMeth=Floor
  Divide1 : Product  Inputs=**  OutDataTypeStr=Inherit: Inherit via back propagation  RndMeth=Simplest
  Switch : Switch  Criteria=u2 ~= 0  SaturateOnIntegerOverflow=off  InputSameDT=off
  Switch1 : Switch  Criteria=u2 ~= 0  OutDataTypeStr=Inherit: Inherit via back propagation  SaturateOnIntegerOverflow=off  InputSameDT=off
  lib_Conversion_1 : lib_conversion/lib_Conversion_0  Commented=on  lb_parDataType=fixdt(1,32)  lb_parOutpMaxVal=lb_parMaxInpVal  lb_parOutpMinVal=lb_parMinInpVal  lb_parSatFlag=off
  lib_ResettableUnitDelay_1 : lib_resettable_unit_delay/lib_ResettableUnitDelay_0
  lb_genIncrOutp : Outport
  lb_genDelyOutp : Outport  Port=2
  wires:
  lb_bolRset/1 -> [lb_bolRset]
  [lb_genDelyOutp] -> lb_genDelyOutp/1
  lb_genInp/1 -> [lb_genInp]
  Constant4/1 -> Divide1/2
  Divide1/1 -> Data Type Conversion/1, Data Type Duplicate/1
  [lb_bolRset] -> lib_ResettableUnitDelay_1/3
  lb_noRatLimReq/1 -> Switch1/2
  lb_incrRatLimReq/1 -> Switch/2
  Constant/1 -> Data Type Duplicate1/1, Switch1/1
  Switch/1 -> Data Type Duplicate1/2, Switch1/3
  Constant2/1 -> Switch/1
  Switch1/1 -> Data Type Duplicate1/3, [lb_trigRateLim]
  Constant1/1 -> Switch/3
  [lb_trigRateLim] -> Divide1/1
  Data Type Conversion/1 -> Add1/1, Data Type Duplicate/2  "lb_incrVal"
  lib_ResettableUnitDelay_1/1 -> Add1/2, [lb_genDelyOutp]
  Add1/1 -> lb_genIncrOutp/1, lib_ResettableUnitDelay_1/1
  [lb_genInp] -> lib_ResettableUnitDelay_1/2  "lb_genIncrInitCond"

== system vhit_control_library/lib_RateLimiter_YXQ_0/sss_DecrementFlagTrigger ==
  lb_genInp : Inport
  lb_genDelyOutp : Inport  Port=2
  Add : Sum  Inputs=+-  OutDataTypeStr=Inherit: Inherit via back propagation  RndMeth=Simplest
  Constant : Constant  OutDataTypeStr=uint16
  Constant1 : Constant  Value=lb_parFallSlewRate
  Constant2 : Constant  Value=lb_parSampTime
  Data Type Duplicate : DataTypeDuplicate
  Data Type Conversion : DataTypeConversion  SaturateOnIntegerOverflow=off  RndMeth=Floor
  Divide1 : Product  Inputs=*/  OutDataTypeStr=Inherit: Inherit via back propagation  RndMeth=Simplest
  Equal : RelationalOperator  Operator=<=  OutDataTypeStr=boolean  RndMeth=Simplest  InputSameDT=off
  Equal1 : RelationalOperator  Operator=<=  OutDataTypeStr=boolean  RndMeth=Simplest  InputSameDT=off
  Logical Operator : Logic  AllPortsSameDT=off  OutDataTypeStr=boolean
  Product : Product  OutDataTypeStr=Inherit: Inherit via back propagation
  lib_Conversion_1 : lib_conversion/lib_Conversion_0  lb_parDataType=fixdt(1,32)  lb_parOutpMaxVal=lb_parInpVrntMaxVal  lb_parOutpMinVal=[]  lb_parSatFlag=off
  lib_Conversion_2 : lib_conversion/lib_Conversion_0  lb_parDataType=lb_parInpDrvtDataType  lb_parOutpMaxVal=lb_parInpDrvtMaxVal  lb_parOutpMinVal=[]  lb_parSatFlag=off
  lib_Conversion_3 : lib_conversion/lib_Conversion_0  lb_parDataType=fixdt(0,32)  lb_parOutpMaxVal=1/double(lb_parSampTime)  lb_parOutpMinVal=[]  lb_parSatFlag=off
  lb_decrRatLimOn : Outport
  wires:
  [lb_genInp] -> Equal/1
  Equal/1 -> Logical Operator/2
  Product/1 -> lib_Conversion_2/1
  Equal1/1 -> Logical Operator/1
  Logical Operator/1 -> lb_decrRatLimOn/1
  lb_genInp/1 -> [lb_genInp]
  lb_genDelyOutp/1 -> [lb_genDelyOutp]
  Constant1/1 -> Data Type Conversion/1
  [lb_genDelyOutp] -> Add/2
  [lb_genDelyOutp] -> Equal/2
  lib_Conversion_2/1 -> Data Type Duplicate/1, Equal1/1  "lb_incrRate"
  [lb_genInp] -> Add/1
  Add/1 -> lib_Conversion_1/1
  lib_Conversion_1/1 -> Product/1  "lb_incrInpVrnt"
  Constant/1 -> Divide1/1
  Constant2/1 -> Divide1/2
  Divide1/1 -> lib_Conversion_3/1
  lib_Conversion_3/1 -> Product/2  "lb_sampTimeInv"
  Data Type Conversion/1 -> Data Type Duplicate/2, Equal1/2

== system vhit_control_library/lib_RateLimiter_YXQ_0/sss_IncrementFlagTrigger ==
  lb_genInp : Inport
  lb_genDelyOutp : Inport  Port=2
  Add : Sum  Inputs=+-  OutDataTypeStr=Inherit: Inherit via back propagation  RndMeth=Simplest
  Constant : Constant  OutDataTypeStr=uint16
  Constant1 : Constant  Value=lb_parRiseSlewRate
  Constant2 : Constant  Value=lb_parSampTime
  Data Type Duplicate : DataTypeDuplicate
  Data Type Conversion : DataTypeConversion  SaturateOnIntegerOverflow=off  RndMeth=Floor
  Divide1 : Product  Inputs=*/  OutDataTypeStr=Inherit: Inherit via back propagation  RndMeth=Simplest
  Equal : RelationalOperator  OutDataTypeStr=boolean  RndMeth=Simplest  InputSameDT=off
  Equal1 : RelationalOperator  OutDataTypeStr=boolean  RndMeth=Simplest  InputSameDT=off
  Logical Operator : Logic  AllPortsSameDT=off  OutDataTypeStr=boolean
  Product : Product  OutDataTypeStr=Inherit: Inherit via back propagation
  lib_Conversion_1 : lib_conversion/lib_Conversion_0  lb_parDataType=fixdt(1,32)  lb_parOutpMaxVal=lb_parInpVrntMaxVal  lb_parOutpMinVal=[]  lb_parSatFlag=off
  lib_Conversion_2 : lib_conversion/lib_Conversion_0  lb_parDataType=lb_parInpDrvtDataType  lb_parOutpMaxVal=lb_parInpDrvtMaxVal  lb_parOutpMinVal=[]  lb_parSatFlag=off
  lib_Conversion_3 : lib_conversion/lib_Conversion_0  lb_parDataType=fixdt(0,32)  lb_parOutpMaxVal=1/double(lb_parSampTime)  lb_parOutpMinVal=[]  lb_parSatFlag=off
  lb_incrRatLimOn : Outport
  wires:
  Add/1 -> lib_Conversion_1/1
  [lb_genInp] -> Equal/1
  Equal/1 -> Logical Operator/2
  Equal1/1 -> Logical Operator/1
  Logical Operator/1 -> lb_incrRatLimOn/1
  lb_genInp/1 -> [lb_genInp]
  lb_genDelyOutp/1 -> [lb_genDelyOutp]
  Product/1 -> lib_Conversion_2/1
  Constant1/1 -> Data Type Conversion/1
  [lb_genDelyOutp] -> Add/2
  [lb_genDelyOutp] -> Equal/2
  lib_Conversion_2/1 -> Data Type Duplicate/1, Equal1/1  "lb_incrRate"
  [lb_genInp] -> Add/1
  lib_Conversion_1/1 -> Product/1  "lb_incrInpVrnt"
  Divide1/1 -> lib_Conversion_3/1
  Constant2/1 -> Divide1/2
  Constant/1 -> Divide1/1
  lib_Conversion_3/1 -> Product/2  "lb_sampTimeInv"
  Data Type Conversion/1 -> Equal1/2, Data Type Duplicate/2

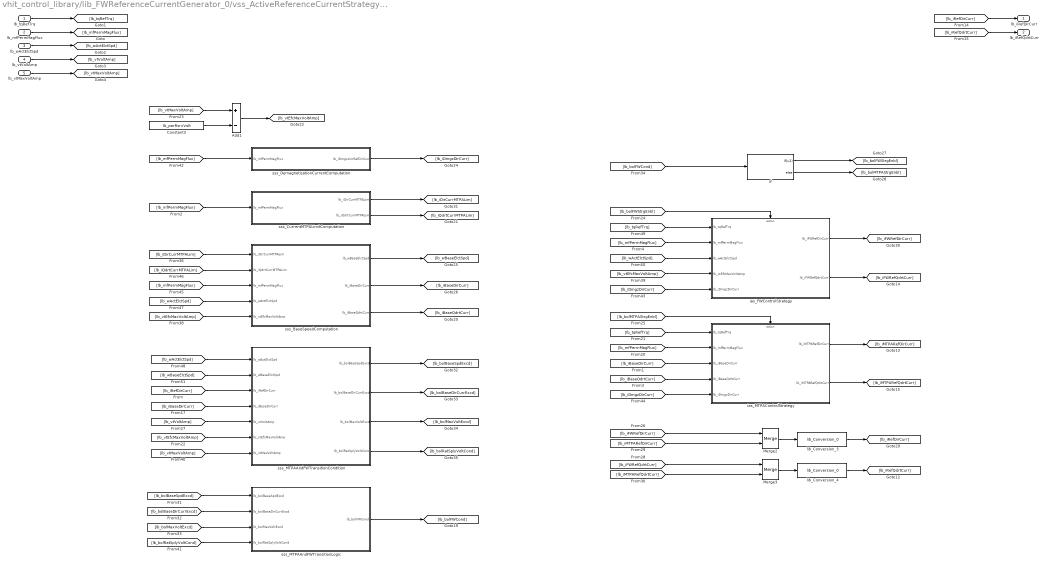
== system vhit_control_library/lib_FWReferenceCurrentGenerator_0/vss_ActiveReferenceCurrentStrategy/vss_FieldWeakeningStrategy ==
  lb_tqRefTrq : Inport
  lb_mfPermMagFlux : Inport  Port=2
  lb_wActElctSpd : Inport  Port=3
  lb_vtVoltAmp : Inport  Port=4
  lb_vtMaxVoltAmp : Inport  Port=5
  Add1 : Sum  Inputs=+-  OutDataTypeStr=Inherit: Same as first input
  Constant3 : Constant  Value=lb_parRsrvVolt
  If : If  IfExpression=u1
  Merge2 : Merge
  Merge3 : Merge
  ias_FWControlStrategy : Subsystem  TreatAsAtomicUnit=on
  ias_MTPAControlStrategy : Subsystem  TreatAsAtomicUnit=on
  lib_Conversion_3 : lib_conversion/lib_Conversion_0  lb_parDataType=lb_parOutpDataType  lb_parOutpMaxVal=[]  lb_parOutpMinVal=[]  lb_parSatFlag=off
  lib_Conversion_4 : lib_conversion/lib_Conversion_0  lb_parDataType=lb_parOutpDataType  lb_parOutpMaxVal=[]  lb_parOutpMinVal=[]  lb_parSatFlag=off
  sss_BaseSpeedComputation : Subsystem
  sss_CurrentMTPALimitComputation : Subsystem
  sss_DemagnetizationCurrentComputation : Subsystem
  sss_MTPAAndFWTransitionCondition : Subsystem
  sss_MTPAAndFWTransitionLogic : Subsystem
  lb_iRefDirCurr : Outport
  lb_iRefQdrtCurr : Outport  Port=2
  wires:
  Merge3/1 -> lib_Conversion_4/1
  [lb_bolFWCond] -> If/1
  [lb_bolMTPAStrgEnbl] -> ias_MTPAControlStrategy/Action
  [lb_iFWRefDirCurr] -> Merge2/1
  [lb_iBaseQdrtCurr] -> ias_MTPAControlStrategy/4(lb_iBaseQdrtCurr)
  [lb_iDmgzDirCurr] -> ias_MTPAControlStrategy/5(lb_iDmgzDirCurr)
  [lb_vtVoltAmp] -> sss_MTPAAndFWTransitionCondition/5(lb_vtVoltAmp)
  [lb_mfPermMagFlux] -> ias_FWControlStrategy/2(lb_mfPermMagFlux)
  [lb_mfPermMagFlux] -> ias_MTPAControlStrategy/2(lb_mfPermMagFlux)
  sss_DemagnetizationCurrentComputation/1(lb_iDmgzLimRefDirCurr) -> [lb_iDmgzDirCurr]
  [lb_bolRatSplyVoltCond] -> sss_MTPAAndFWTransitionLogic/4(lb_bolRatSplyVoltCond)
  [lb_bolBaseSpdExcd] -> sss_MTPAAndFWTransitionLogic/1(lb_bolBaseSpdExcd)
  [lb_bolBaseDirCurrExcd] -> sss_MTPAAndFWTransitionLogic/2(lb_bolBaseDirCurrExcd)
  lib_Conversion_4/1 -> [lb_iRefQdrtCurr]
  [lb_wActElctSpd] -> ias_FWControlStrategy/3(lb_wActElctSpd)
  ias_MTPAControlStrategy/1(lb_iMTPARefDirCurr) -> [lb_iMTPARefDirCurr]
  ias_FWControlStrategy/2(lb_iFWRefQdrtCurr) -> [lb_iFWRefQdrtCurr]
  [lb_mfPermMagFlux] -> sss_CurrentMTPALimitComputation/1(lb_mfPermMagFlux)
  [lb_iQdrtCurrMTPALim] -> sss_BaseSpeedComputation/2(lb_iQdrtCurrMTPALim)
  [lb_iBaseDirCurr] -> sss_MTPAAndFWTransitionCondition/4(lb_iBaseDirCurr)
  [lb_vtMaxVoltAmp] -> Add1/1
  Add1/1 -> [lb_vtEfcMaxVoltAmp]
  [lb_bolFWStrgEnbl] -> ias_FWControlStrategy/Action
  sss_BaseSpeedComputation/3(lb_iBaseQdrtCurr) -> [lb_iBaseQdrtCurr]
  Constant3/1 -> Add1/2
  sss_CurrentMTPALimitComputation/1(lb_iDirCurrMTPALim) -> [lb_iDirCurrMTPALim]
  Merge2/1 -> lib_Conversion_3/1
  [lb_iBaseDirCurr] -> ias_MTPAControlStrategy/3(lb_iBaseDirCurr)
  [lb_iRefQdrtCurr] -> lb_iRefQdrtCurr/1
  lb_mfPermMagFlux/1 -> [lb_mfPermMagFlux]
  lb_tqRefTrq/1 -> [lb_tqRefTrq]
  [lb_iDirCurrMTPALim] -> sss_BaseSpeedComputation/1(lb_iDirCurrMTPALim)
  [lb_iRefDirCurr] -> lb_iRefDirCurr/1
  [lb_tqRefTrq] -> ias_FWControlStrategy/1(lb_tqRefTrq)
  [lb_mfPermMagFlux] -> sss_BaseSpeedComputation/3(lb_mfPermMagFlux)
  lb_vtVoltAmp/1 -> [lb_vtVoltAmp]
  sss_MTPAAndFWTransitionCondition/4(lb_bolRatSplyVoltCond) -> [lb_bolRatSplyVoltCond]
  [lb_iMTPARefDirCurr] -> Merge2/2
  sss_MTPAAndFWTransitionCondition/3(lb_bolMaxVoltExcd) -> [lb_bolMaxVoltExcd]
  sss_CurrentMTPALimitComputation/2(lb_iQdrtCurrMTPALim) -> [lb_iQdrtCurrMTPALim]
  [lb_vtEfcMaxVoltAmp] -> sss_MTPAAndFWTransitionCondition/6(lb_vtEfcMaxVoltAmp)
  [lb_wBaseElctSpd] -> sss_MTPAAndFWTransitionCondition/2(lb_wBaseElctSpd)
  ias_MTPAControlStrategy/2(lb_iMTPARefQdrtCurr) -> [lb_iMTPARefQdrtCurr]
  lib_Conversion_3/1 -> [lb_iRefDirCurr]
  [lb_vtMaxVoltAmp] -> sss_MTPAAndFWTransitionCondition/7(lb_vtMaxVoltAmp)
  [lb_wActElctSpd] -> sss_MTPAAndFWTransitionCondition/1(lb_wActElctSpd)
  lb_vtMaxVoltAmp/1 -> [lb_vtMaxVoltAmp]
  sss_MTPAAndFWTransitionLogic/1(lb_bolFWCond) -> [lb_bolFWCond]
  sss_BaseSpeedComputation/2(lb_iBaseDirCurr) -> [lb_iBaseDirCurr]
  [lb_bolMaxVoltExcd] -> sss_MTPAAndFWTransitionLogic/3(lb_bolMaxVoltExcd)
  lb_wActElctSpd/1 -> [lb_wActElctSpd]
  [lb_iRefDirCurr] -> sss_MTPAAndFWTransitionCondition/3(lb_iRefDirCurr)
  sss_BaseSpeedComputation/1(lb_wBaseElctSpd) -> [lb_wBaseElctSpd]
  sss_MTPAAndFWTransitionCondition/2(lb_bolBaseDirCurrExcd) -> [lb_bolBaseDirCurrExcd]
  ias_FWControlStrategy/1(lb_iFWRefDirCurr) -> [lb_iFWRefDirCurr]
  [lb_tqRefTrq] -> ias_MTPAControlStrategy/1(lb_tqRefTrq)
  [lb_wActElctSpd] -> sss_BaseSpeedComputation/4(lb_wActElctSpd)
  [lb_mfPermMagFlux] -> sss_DemagnetizationCurrentComputation/1(lb_mfPermMagFlux)
  If/2 -> [lb_bolMTPAStrgEnbl]
  [lb_vtEfcMaxVoltAmp] -> sss_BaseSpeedComputation/5(lb_vtEfcMaxVoltAmp)
  [lb_iDmgzDirCurr] -> ias_FWControlStrategy/5(lb_iDmgzDirCurr)
  [lb_vtEfcMaxVoltAmp] -> ias_FWControlStrategy/4(lb_vtEfcMaxVoltAmp)
  [lb_iFWRefQdrtCurr] -> Merge3/1
  sss_MTPAAndFWTransitionCondition/1(lb_bolBaseSpdExcd) -> [lb_bolBaseSpdExcd]
  [lb_iMTPARefQdrtCurr] -> Merge3/2
  If/1 -> [lb_bolFWStrgEnbl]

== system vhit_control_library/lib_FWReferenceCurrentGenerator_0/vss_ActiveReferenceCurrentStrategy/vss_MaximumTorquePerAmpereStrategy ==
  lb_tqRefTrq : Inport
  lb_mfPermMagFlux : Inport  Port=2
  ias_MTPAControlStrategy : Subsystem  TreatAsAtomicUnit=on
  sss_CurrentMTPALimitComputation : Subsystem
  sss_DemagnetizationCurrentComputation : Subsystem
  lb_iRefDirCurr : Outport
  lb_iRefQdrtCurr : Outport  Port=2
  wires:
  ias_MTPAControlStrategy/2(lb_iRefQdrtCurr) -> [lb_iRefQdrtCurr]
  ias_MTPAControlStrategy/1(lb_iRefDirCurr) -> [lb_iRefDirCurr]
  [lb_iQdrtCurrMTPALim] -> ias_MTPAControlStrategy/4(lb_iQdrtCurrMTPALim)
  [lb_iDmgzDirCurr] -> ias_MTPAControlStrategy/5(lb_iDmgzDirCurr)
  [lb_mfPermMagFlux] -> ias_MTPAControlStrategy/2(lb_mfPermMagFlux)
  sss_DemagnetizationCurrentComputation/1(lb_iDmgzLimRefDirCurr) -> [lb_iDmgzDirCurr]
  sss_CurrentMTPALimitComputation/2(lb_iQdrtCurrMTPALim) -> [lb_iQdrtCurrMTPALim]
  [lb_mfPermMagFlux] -> sss_CurrentMTPALimitComputation/1(lb_mfPermMagFlux)
  lb_mfPermMagFlux/1 -> [lb_mfPermMagFlux]
  [lb_iRefDirCurr] -> lb_iRefDirCurr/1
  [lb_tqRefTrq] -> ias_MTPAControlStrategy/1(lb_tqRefTrq)
  sss_CurrentMTPALimitComputation/1(lb_iDirCurrMTPALim) -> [lb_iDirCurrMTPALim]
  lb_tqRefTrq/1 -> [lb_tqRefTrq]
  [lb_iRefQdrtCurr] -> lb_iRefQdrtCurr/1
  [lb_iDirCurrMTPALim] -> ias_MTPAControlStrategy/3(lb_iDirCurrMTPALim)
  [lb_mfPermMagFlux] -> sss_DemagnetizationCurrentComputation/1(lb_mfPermMagFlux)
